simulink model "input output linearization"  (R2020a)
settings: Solver=VariableStepAuto  StartTime=0.0  StopTime=10  RelTol=1e-3
values from neighbouring files (symbols this model uses):
  b = 0.04    [Cubic_cartesian_polynomial.m]
settings Model: Creator=ThinkPad  LastModifiedBy=ThinkPad

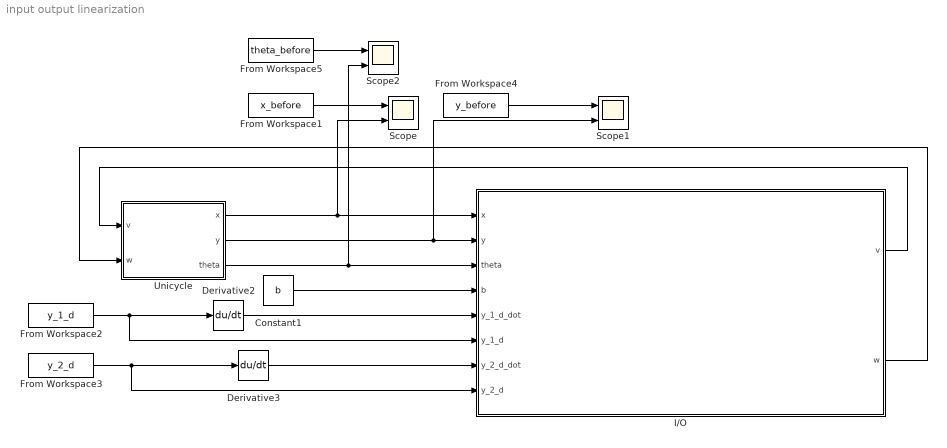
== system input output linearization ==
  Constant1 : Constant  Value=b
  Derivative2 : Derivative
  Derivative3 : Derivative
  From Workspace1 : FromWorkspace  VariableName=x_before  SampleTime=-1  OutputAfterFinalValue=Holding final value
  From Workspace2 : FromWorkspace  VariableName=y_1_d  SampleTime=-1  OutputAfterFinalValue=Holding final value
  From Workspace3 : FromWorkspace  VariableName=y_2_d  SampleTime=-1  OutputAfterFinalValue=Holding final value
  From Workspace4 : FromWorkspace  VariableName=y_before  SampleTime=-1  OutputAfterFinalValue=Holding final value
  From Workspace5 : FromWorkspace  VariableName=theta_before  SampleTime=-1  OutputAfterFinalValue=Holding final value
  I/O : Subsystem
  Scope : Scope  NumInputPorts=2
  Scope1 : Scope  NumInputPorts=2
  Scope2 : Scope  NumInputPorts=2
  Unicycle : Subsystem
  wires:
  From Workspace2/1 -> I/O/6(y_1_d), Derivative2/1
  I/O/1(v) -> Unicycle/1(v)
  Unicycle/3(theta) -> Scope2/2, I/O/3(theta)
  Derivative2/1 -> I/O/5(y_1_d_dot)
  From Workspace3/1 -> I/O/8(y_2_d), Derivative3/1
  Derivative3/1 -> I/O/7(y_2_d_dot)
  I/O/2(w) -> Unicycle/2(w)
  Unicycle/1(x) -> I/O/1(x), Scope/2
  Constant1/1 -> I/O/4(b)
  Unicycle/2(y) -> Scope1/2, I/O/2(y)
  From Workspace1/1 -> Scope/1
  From Workspace4/1 -> Scope1/1
  From Workspace5/1 -> Scope2/1

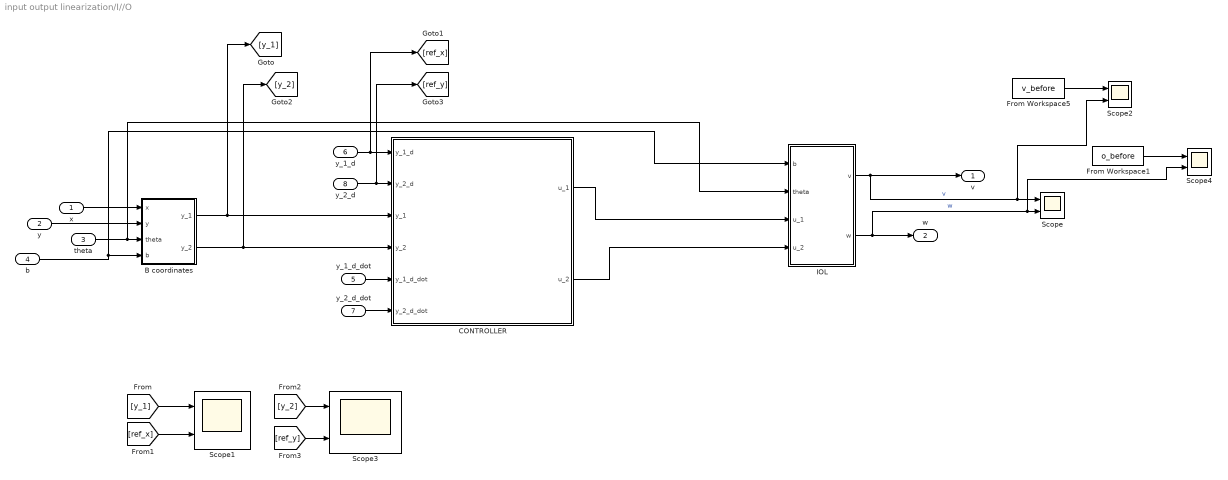
== system input output linearization/I//O ==
  x : Inport
  y : Inport  Port=2
  theta : Inport  Port=3
  b : Inport  Port=4
  y_1_d_dot : Inport  Port=5
  y_1_d : Inport  Port=6
  y_2_d_dot : Inport  Port=7
  y_2_d : Inport  Port=8
  B coordinates : MATLAB Function  TreatAsAtomicUnit=on
  CONTROLLER : MATLAB Function  TreatAsAtomicUnit=on
  From Workspace1 : FromWorkspace  VariableName=o_before  SampleTime=-1  OutputAfterFinalValue=Holding final value
  From Workspace5 : FromWorkspace  VariableName=v_before  SampleTime=-1  OutputAfterFinalValue=Holding final value
  IOL : MATLAB Function  TreatAsAtomicUnit=on
  Scope{,1..4} (5 alike) : Scope  NumInputPorts=2
  v : Outport
  w : Outport  Port=2
  wires:
  theta/1 -> IOL/2(theta), B coordinates/3(theta)
  y_2_d_dot/1 -> CONTROLLER/6(y_2_d_dot)
  B coordinates/1(y_1) -> CONTROLLER/3(y_1), [y_1]
  y_2_d/1 -> [ref_y], CONTROLLER/2(y_2_d)
  CONTROLLER/1(u_1) -> IOL/3(u_1)
  b/1 -> IOL/1(b), B coordinates/4(b)
  y/1 -> B coordinates/2(y)
  B coordinates/2(y_2) -> [y_2], CONTROLLER/4(y_2)
  y_1_d_dot/1 -> CONTROLLER/5(y_1_d_dot)
  CONTROLLER/2(u_2) -> IOL/4(u_2)
  y_1_d/1 -> [ref_x], CONTROLLER/1(y_1_d)
  IOL/2(w) -> w/1, Scope4/2, Scope/2  "w"
  x/1 -> B coordinates/1(x)
  IOL/1(v) -> v/1, Scope2/2, Scope/1  "v"
  [y_1] -> Scope1/1
  [ref_x] -> Scope1/2
  [y_2] -> Scope3/1
  [ref_y] -> Scope3/2
  From Workspace5/1 -> Scope2/1
  From Workspace1/1 -> Scope4/1

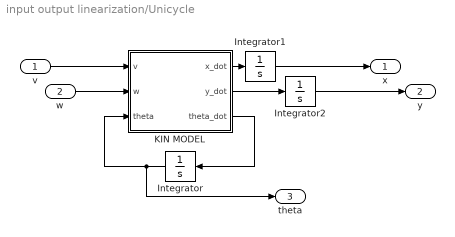
== system input output linearization/Unicycle ==
  v : Inport
  w : Inport  Port=2
  Integrator : Integrator
  Integrator1 : Integrator
  Integrator2 : Integrator
  KIN MODEL : MATLAB Function  TreatAsAtomicUnit=on
  x : Outport
  y : Outport  Port=2
  theta : Outport  Port=3
  wires:
  KIN MODEL/1(x_dot) -> Integrator1/1
  v/1 -> KIN MODEL/1(v)
  KIN MODEL/2(y_dot) -> Integrator2/1
  Integrator/1 -> theta/1, KIN MODEL/3(theta)
  Integrator1/1 -> x/1
  w/1 -> KIN MODEL/2(w)
  Integrator2/1 -> y/1
  KIN MODEL/3(theta_dot) -> Integrator/1

== matlab function input output linearization/I//O/B coordinates ==
  data: x input; y_1 output; y input; theta input; b input; y_2 output
function [y_1,y_2] = fcn(x,y,theta,b)
y_1=x+b*cos(theta);
y_2=y+b*sin(theta);

== matlab function input output linearization/I//O/CONTROLLER ==
  data: y_1_d input; u_1 output; y_2_d input; y_1 input; y_2 input; y_1_d_dot input; y_2_d_dot input; u_2 output
function [u_1,u_2] = fcn(y_1_d,y_2_d,y_1,y_2,y_1_d_dot,y_2_d_dot)
k_1=2;
k_2=2;
u_1=y_1_d_dot+k_1*(y_1_d-y_1);
u_2=y_2_d_dot+k_2*(y_2_d-y_2);

== matlab function input output linearization/I//O/IOL ==
  data: b input; theta input; v output; w output; u_1 input; u_2 input
function [v,w] = fcn(b,theta,u_1,u_2)
T=[ cos(theta),  -b*sin(theta);
    sin(theta),  b*cos(theta)];
T_inv=inv(T);
v=T_inv(1,:)*[u_1;u_2];
w=T_inv(2,:)*[u_1;u_2];

== matlab function input output linearization/Unicycle/KIN MODEL ==
  data: v input; x_dot output; w input; y_dot output; theta_dot output; theta input
function [x_dot,y_dot,theta_dot] = fcn(v,w,theta)
x_dot=cos(theta)*v
y_dot=sin(theta)*v
theta_dot=w;
